simulink model "top_level_57_ALL_bergeron"  (R2025b)
settings: Solver=FixedStepDiscrete  StartTime=0.0  StopTime=50  FixedStep=Ts  RelTol=1e-3
undefined symbols (not defined in the file): DiscIntNeverNeededParam, droop, genTrip, idxGenTrip, idxSG_01, idxSMa, idxSMb, n_genP_pu, n_vRef_pu, noSG, noSM, Pref_lock, rateV, tagI, Ts, wref
libraries: simulink x4, ee_lib_for_power_systems x2, eeGeneralControl x1, eeSinusoidalMeasurementV2 x1
settings Model: SimulationMode=accelerator  Creator=gdudgeon  LastModifiedBy=gdudgeon
settings DataIOCC: SaveOutput=off  DSMLogging=off  InspectSignalLogs=on  SaveTime=off
settings ModelReferenceCC: UpdateModelReferenceTargets=AssumeUpToDate  ParallelModelReferenceMATLABWorkerInit=Copy Base Workspace

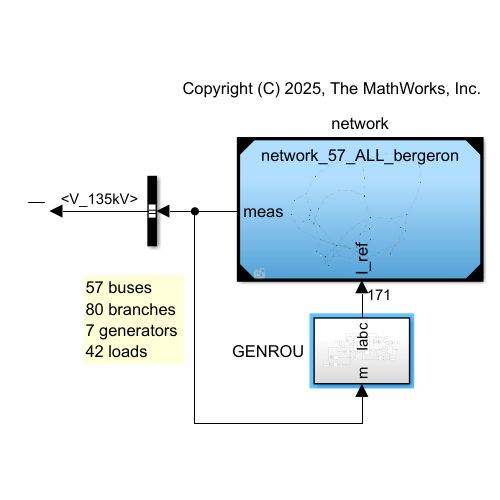
[thumbnail: Simulink's stored preview of the top-level diagram]
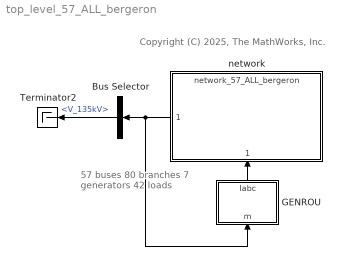
== system top_level_57_ALL_bergeron ==
  note: 57 buses
      | 80 branches
      | 7 generators
      | 42 loads
  note: Copyright (C) 2025, The MathWorks, Inc.
  Bus Selector : BusSelector  OutputSignals=V_135kV
  GENROU : Subsystem
  Terminator2 : Terminator
  network : ModelReference  ModelNameDialog=network_57_ALL_bergeron  ModelReferenceVersion=5.1
      settings: PortSchema="{\"entries\":[{\"content\":{\"sides\":[{\"content\":{\"connectorIds\":[\"Out1\"]},\"type\":\"ConnectorPlacement.EquallySpacedRectSide\",\"uuid\":\"a74df316-1767-4f8a-840d-17e03cd258f4\"},{\"content\":{\"side\":\"RIGHT\"},\"type\":\"ConnectorPlacement.EquallySpacedRectSide\",\"uuid\":\"1b3c021f-69ce-4b13-aefa-cee96e0614ce\"},{\"content\":{\"side\":\"TOP\"},\"type\":\"ConnectorPlacement.EquallySpacedRectSide\",\"uuid\":\"ae15f7f3-c1e2-4a2f-99df-e8d2d0ffd4ae\"},{\"content\":{\"connectorIds\":[\"In1\"],\"side\":\"BOTTOM\"},\"type\":\"ConnectorPlacement.EquallySpacedRectSide\",\"uuid\":\"649ce0cc-47ac-44c8-b67b-0ed46c10a575\"}]},\"type\":\"ConnectorPlacement.EquallySpacedConnector\",\"uuid\":\"f8de1fa7-a54d-42cb-bb68-f09d9f668e45\"}],\"packageUris\":[\"http://schema.mathworks.com/mf0/Connector/R2020b\"],\"version\":\"1.0\"}"
  wires:
  GENROU/1(Iabc) -> network/1
  network/1 -> Bus Selector/1, GENROU/1(m)
  Bus Selector/1 -> Terminator2/1  "<V_135kV>"

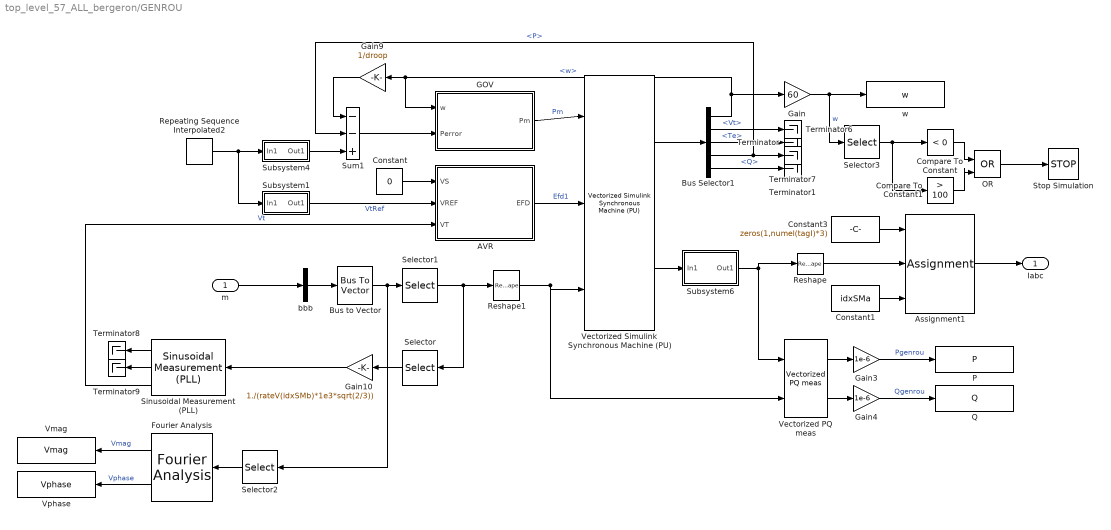
== system top_level_57_ALL_bergeron/GENROU ==
  m : Inport
  AVR : Subsystem  mask{K=500*ones(1,numel(idxSMb)), TE=0.05*ones(1,numel(idxSMb)), EMIN=0*ones(1,numel(idxSMb)), EMAX=4*ones(1,numel(idxSMb))}
      mask Display: disp('AVR')
  Assignment1 : Assignment  IndexOptions=Index vector (port)  Indices=1  OutputSizes=1
  Bus Selector1 : BusSelector  OutputSignals=w,Vt,Te,P,Q
  Bus to Vector : BusToVector
  Compare To Constant : simulink/Logic and Bit Operations/Compare To Constant  relop=<  const=0  OutDataTypeStr=boolean
  Compare To Constant1 : simulink/Logic and Bit Operations/Compare To Constant  relop=>  const=100  OutDataTypeStr=boolean
  Constant : Constant  Value=0  SampleTime=Ts
  Constant1 : Constant  Value=idxSMa  SampleTime=Ts
  Constant3 : Constant  Value=zeros(1,numel(tagI)*3)  SampleTime=Ts
  Fourier Analysis : eeGeneralControl/Fourier Analysis  f=freq  n=1  M0=1  Ph0=0  BufferSize=8192  Ts=Ts
      settings: LibrarySourceBlock=ee_sl_lib/General Control/Fourier Analysis
  GOV : Subsystem
      mask Display: disp('GOV')
  Gain : Gain  Gain=60
  Gain10 : Gain  Gain=1./(rateV(idxSMb)*1e3*sqrt(2/3))
  Gain3 : Gain  Gain=1e-6
  Gain4 : Gain  Gain=1e-6
  Gain9 : Gain  Gain=1/droop
  OR : Logic  Operator=OR  IconShape=distinctive  AllPortsSameDT=off  OutDataTypeStr=boolean
  P : ToWorkspace  VariableName=P  SaveFormat=Timeseries  SampleTime=Ts
  Q : ToWorkspace  VariableName=Q  SaveFormat=Timeseries  SampleTime=Ts
  Repeating Sequence Interpolated2 : simulink/Sources/Repeating Sequence Interpolated  OutValues=[0 0 1 1]  TimeValues=[0 0.2 1 110]  LookUpMeth=Interpolation-Use End Values  tsamp=Ts  OutMin=[]  OutMax=[]  OutDataTypeStr=double  OutputDataTypeScalingMode=double  OutDataType=fixdt(0,8)  OutScaling=2^-10
  Reshape : Reshape
  Reshape1 : Reshape  OutputDimensionality=Customize  OutputDimensions=[3,numel(idxSMb)]
  Selector : Selector  InputPortWidth=numel(idxSMb)*3  IndexOptions=Index vector (dialog)  Indices=1:3:numel(idxSMb)*3  OutputSizes=1
  Selector1 : Selector  InputPortWidth=numel(tagI)*3  IndexOptions=Index vector (dialog)  Indices=idxSMa  OutputSizes=1
  Selector2 : Selector  InputPortWidth=57*3  IndexOptions=Index vector (dialog)  Indices=1:3:(57*3)  OutputSizes=1
  Selector3 : Selector  InputPortWidth=noSM  IndexOptions=Index vector (dialog)  Indices=1  OutputSizes=1
  Sinusoidal Measurement (PLL) : eeSinusoidalMeasurementV2/Sinusoidal Measurement (PLL)  Ki_PD=1000  Kp_LF=400  Ki_LF=20000  F0=60  Theta0=0  Mag0=0  Ts=Ts
      settings: LibrarySourceBlock=|
      | ee_sl_lib/Measurements/Sinusoidal Measurement
      | (PLL)
  Stop Simulation : Stop
  Subsystem1 : Subsystem
  Subsystem4 : Subsystem
  Subsystem6 : Subsystem  mask{tn=idxGenTrip}
      mask prompts: tn "Generator index"
      mask Display: disp('TRIP')
  Sum1 : Sum  Inputs=--+
  Terminator{,1,6..9} (6 alike) : Terminator
  Vectorized PQ meas : ee_lib_for_power_systems/Sense and Measure/Vectorized PQ meas  SystemSampleTime=-1  VariantActivationTime=update diagram  EmptyChoice=off  PassThrough=off  PassThroughVariantControl=(default)  EmptyChoiceVariantControl=(default)  AllowFlexibleInterface=on  Latency=0  AutoFrameSizeCalculation=off
      settings: LibrarySourceBlock=|
      | sps_lib/Sensors and Measurements/Power
      | (3ph, Instantaneous)
  Vectorized Simulink Synchronous Machine (PU) : ee_lib_for_power_systems/Electromechanical Machines/Vectorized Simulink Synchronous Machine (PU)  Pnom=nomP_SM  Vnom=rateV(idxSMb)*1e3  fnom=60*ones(1,noSM)  NPP=4*ones(1,noSM)  Ra=0.05*ones(1,noSM)  Xl=0.1*ones(1,noSM)  Xd=1.5*ones(1,noSM)  Xq=1.4*ones(1,noSM)  Xdp=0.4*ones(1,noSM)  Xqp=0.5*ones(1,noSM)  Xdpp=0.25*ones(1,noSM)  Xqpp=0.25*ones(1,noSM)  Tdop=5*ones(1,noSM)  Tqop=1.5*ones(1,noSM)  Tdopp=0.6*ones(1,noSM)  Tqopp=0.06*ones(1,noSM)  H=4*ones(1,noSM)  D=zeros(1,noSM)  SatX=SatX  xVec=xVec  no_gens=noSM
      settings: SourceProductName=Support Library for Power Systems
  Vmag : ToWorkspace  VariableName=Vmag  SaveFormat=Timeseries  SampleTime=Ts
  Vphase : ToWorkspace  VariableName=Vphase  SaveFormat=Timeseries  SampleTime=Ts
  bbb : BusSelector  OutputSignals=V_135kV  OutputAsBus=on
  w : ToWorkspace  VariableName=w  SaveFormat=Timeseries  SampleTime=Ts
  Iabc : Outport
  wires:
  Gain3/1 -> P/1  "Pgenrou"
  Vectorized PQ meas/1 -> Gain3/1
  Vectorized PQ meas/2 -> Gain4/1
  Gain4/1 -> Q/1  "Qgenrou"
  Bus Selector1/3 -> Terminator/1  "<Te>"
  Vectorized Simulink Synchronous Machine (PU)/1 -> Bus Selector1/1
  Reshape1/1 -> Vectorized Simulink Synchronous Machine (PU)/3, Vectorized PQ meas/2
  Vectorized Simulink Synchronous Machine (PU)/2 -> Subsystem6/1(In1)
  Constant3/1 -> Assignment1/1
  Constant1/1 -> Assignment1/3
  Assignment1/1 -> Iabc/1
  Repeating Sequence Interpolated2/1 -> Subsystem1/1(In1), Subsystem4/1(In1)
  Reshape/1 -> Assignment1/2
  Subsystem6/1(Out1) -> Vectorized PQ meas/1, Reshape/1
  Bus Selector1/5 -> Terminator1/1  "<Q>"
  Bus Selector1/2 -> Terminator6/1  "<Vt>"
  Bus Selector1/1 -> Gain/1, GOV/1(w), Gain9/1  "<w>"
  Bus Selector1/4 -> Sum1/2, Terminator7/1  "<P>"
  Sum1/1 -> GOV/2(Perror)
  Selector/1 -> Gain10/1
  Sinusoidal Measurement (PLL)/3 -> AVR/3(VT)  "Vt"
  Gain10/1 -> Sinusoidal Measurement (PLL)/1
  Sinusoidal Measurement (PLL)/1 -> Terminator8/1
  Sinusoidal Measurement (PLL)/2 -> Terminator9/1
  Gain9/1 -> Sum1/1
  Subsystem1/1(Out1) -> AVR/2(VREF)  "VtRef"
  Subsystem4/1(Out1) -> Sum1/3
  Gain/1 -> Selector3/1, w/1  "w"
  Constant/1 -> AVR/1(VS)
  m/1 -> bbb/1
  bbb/1 -> Bus to Vector/1
  Selector1/1 -> Selector/1, Reshape1/1
  GOV/1(Pm) -> Vectorized Simulink Synchronous Machine (PU)/1  "Pm"
  AVR/1(EFD) -> Vectorized Simulink Synchronous Machine (PU)/2  "Efd1"
  Fourier Analysis/1 -> Vmag/1  "Vmag"
  Fourier Analysis/2 -> Vphase/1  "Vphase"
  Selector2/1 -> Fourier Analysis/1
  Bus to Vector/1 -> Selector2/1, Selector1/1
  Selector3/1 -> Compare To Constant1/1, Compare To Constant/1
  Compare To Constant/1 -> OR/1
  Compare To Constant1/1 -> OR/2
  OR/1 -> Stop Simulation/1

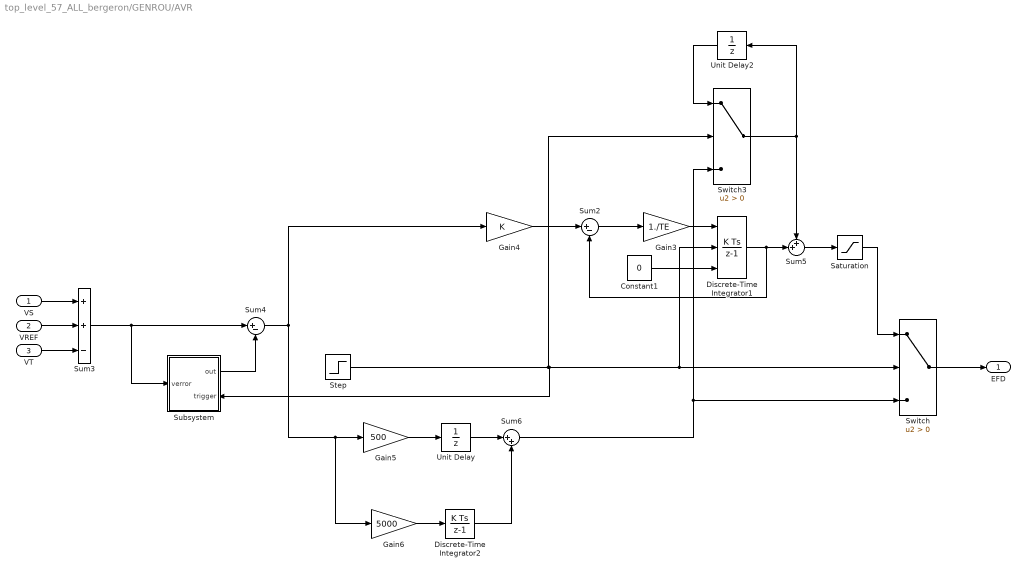
== system top_level_57_ALL_bergeron/GENROU/AVR ==
  VS : Inport
  VREF : Inport  Port=2
  VT : Inport  Port=3
  Constant1 : Constant  Value=0  SampleTime=Ts
  Discrete-Time Integrator1 : DiscreteIntegrator  ExternalReset=rising  InitialConditionSource=external  SampleTime=Ts  UpperSaturationLimit=EMAX  LowerSaturationLimit=EMIN  ICPrevOutput=DiscIntNeverNeededParam  ICPrevScaledInput=DiscIntNeverNeededParam
  Discrete-Time Integrator2 : DiscreteIntegrator  SampleTime=-1  ICPrevOutput=DiscIntNeverNeededParam  ICPrevScaledInput=DiscIntNeverNeededParam
  Gain3 : Gain  Gain=1./TE
  Gain4 : Gain  Gain=K
  Gain5 : Gain  Gain=500
  Gain6 : Gain  Gain=5000
  Saturation : Saturate  UpperLimit=EMAX  LowerLimit=EMIN
  Step : Step  Time=Pref_lock  SampleTime=Ts
  Subsystem : Subsystem
      settings: PortSchema="{\"entries\":[{\"content\":{\"sides\":[{\"content\":{\"connectorIds\":[\"In1\"]},\"type\":\"ConnectorPlacement.EquallySpacedRectSide\",\"uuid\":\"fcea7782-709e-438a-a641-262ec3f31354\"},{\"content\":{\"connectorIds\":[\"Out1\",\"In2\"],\"side\":\"RIGHT\"},\"type\":\"ConnectorPlacement.EquallySpacedRectSide\",\"uuid\":\"9571ea79-f1f3-4aec-b926-22759d29ebce\"},{\"content\":{\"side\":\"TOP\"},\"type\":\"ConnectorPlacement.EquallySpacedRectSide\",\"uuid\":\"bf0a6030-28c1-4408-9c1d-af564ece2abc\"}]},\"type\":\"ConnectorPlacement.EquallySpacedConnector\",\"uuid\":\"5fd903bf-193d-421d-8000-bea997fdfc71\"}],\"packageUris\":[\"http://schema.mathworks.com/mf0/Connector/R2020b\"],\"version\":\"1.0\"}"
  Sum2 : Sum  Inputs=|+-
  Sum3 : Sum  Inputs=++-
  Sum4 : Sum  Inputs=|+-
  Sum5 : Sum  Inputs=++|
  Sum6 : Sum  Inputs=|++
  Switch : Switch  Criteria=u2 > Threshold  SaturateOnIntegerOverflow=off  InputSameDT=off
  Switch3 : Switch  Criteria=u2 > Threshold  SaturateOnIntegerOverflow=off  InputSameDT=off
  Unit Delay : UnitDelay  SampleTime=Ts  HasFrameUpgradeWarning=on
  Unit Delay2 : UnitDelay  SampleTime=Ts  HasFrameUpgradeWarning=on
  EFD : Outport
  wires:
  VS/1 -> Sum3/1
  VREF/1 -> Sum3/2
  VT/1 -> Sum3/3
  Gain4/1 -> Sum2/1
  Sum2/1 -> Gain3/1
  Gain3/1 -> Discrete-Time Integrator1/1
  Switch/1 -> EFD/1
  Sum6/1 -> Switch3/3, Switch/3
  Step/1 -> Discrete-Time Integrator1/2, Switch/2, Subsystem/2(trigger), Switch3/2
  Discrete-Time Integrator1/1 -> Sum2/2, Sum5/2
  Sum5/1 -> Saturation/1
  Switch3/1 -> Unit Delay2/1, Sum5/1
  Unit Delay2/1 -> Switch3/1
  Constant1/1 -> Discrete-Time Integrator1/3
  Gain5/1 -> Unit Delay/1
  Saturation/1 -> Switch/1
  Gain6/1 -> Discrete-Time Integrator2/1
  Discrete-Time Integrator2/1 -> Sum6/2
  Sum4/1 -> Gain4/1, Gain5/1, Gain6/1
  Unit Delay/1 -> Sum6/1
  Subsystem/1(out) -> Sum4/2
  Sum3/1 -> Subsystem/1(verror), Sum4/1

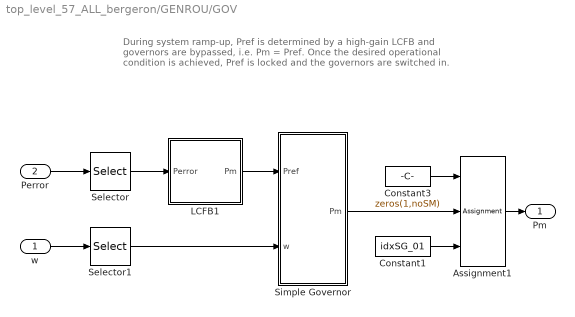
== system top_level_57_ALL_bergeron/GENROU/GOV ==
  note: During system ramp-up, Pref is determined by a high-gain LCFB and governors are bypassed, i.e. Pm = Pref.
      |
      | Once the desired operational condition is achieved, Pref is locked and the governors are switched in.
  w : Inport
  Perror : Inport  Port=2
  Assignment1 : Assignment  IndexOptions=Index vector (port)  Indices=1  OutputSizes=1
  Constant1 : Constant  Value=idxSG_01  SampleTime=Ts
  Constant3 : Constant  Value=zeros(1,noSM)  SampleTime=Ts
  LCFB1 : Subsystem
  Selector : Selector  InputPortWidth=noSM  IndexOptions=Index vector (dialog)  Indices=idxSG_01  OutputSizes=1
  Selector1 : Selector  InputPortWidth=noSM  IndexOptions=Index vector (dialog)  Indices=idxSG_01  OutputSizes=1
  Simple Governor : Subsystem  mask{R=0.2*ones(1,noSG), T1=3*ones(1,noSG), P_MAX=2*ones(1,noSG), P_MIN=0*ones(1,noSG)}
  Pm : Outport
  wires:
  LCFB1/1(Pm) -> Simple Governor/1(Pref)
  Perror/1 -> Selector/1
  w/1 -> Selector1/1
  Simple Governor/1(Pm) -> Assignment1/2
  Constant3/1 -> Assignment1/1
  Constant1/1 -> Assignment1/3
  Assignment1/1 -> Pm/1
  Selector/1 -> LCFB1/1(Perror)
  Selector1/1 -> Simple Governor/2(w)

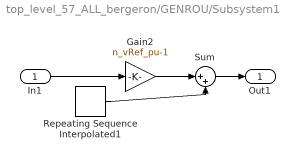
== system top_level_57_ALL_bergeron/GENROU/Subsystem1 ==
  In1 : Inport
  Gain2 : Gain  Gain=n_vRef_pu-1
  Repeating Sequence Interpolated1 : simulink/Sources/Repeating Sequence Interpolated  OutValues=[0 0 1 1]*1  TimeValues=[0 0.05 0.1 110]  LookUpMeth=Interpolation-Use End Values  tsamp=Ts  OutMin=[]  OutMax=[]  OutDataTypeStr=double  OutputDataTypeScalingMode=double  OutDataType=fixdt(0,8)  OutScaling=2^-10
  Sum : Sum  Inputs=|++
  Out1 : Outport
  wires:
  Gain2/1 -> Sum/1
  Repeating Sequence Interpolated1/1 -> Sum/2
  Sum/1 -> Out1/1
  In1/1 -> Gain2/1

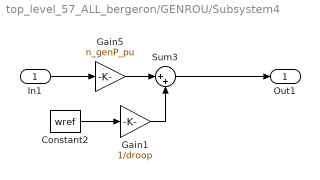
== system top_level_57_ALL_bergeron/GENROU/Subsystem4 ==
  In1 : Inport
  Constant2 : Constant  Value=wref  VectorParams1D=off  SampleTime=Ts
  Gain1 : Gain  Gain=1/droop
  Gain5 : Gain  Gain=n_genP_pu
  Sum3 : Sum  Inputs=|++
  Out1 : Outport
  wires:
  Sum3/1 -> Out1/1
  Gain1/1 -> Sum3/2
  Gain5/1 -> Sum3/1
  In1/1 -> Gain5/1
  Constant2/1 -> Gain1/1

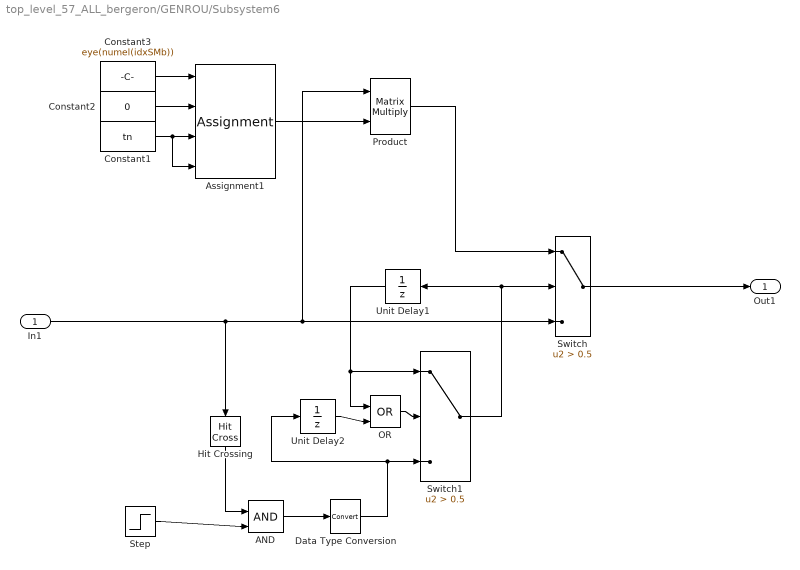
== system top_level_57_ALL_bergeron/GENROU/Subsystem6 ==
  In1 : Inport
  AND : Logic  IconShape=distinctive  AllPortsSameDT=off  OutDataTypeStr=boolean
  Assignment1 : Assignment  NumberOfDimensions=2  IndexOptions=Index vector (port),Index vector (port)  Indices=1,1  OutputSizes=1,1
  Constant1 : Constant  Value=tn  SampleTime=Ts
  Constant2 : Constant  Value=0  SampleTime=Ts
  Constant3 : Constant  Value=eye(numel(idxSMb))  VectorParams1D=off  SampleTime=Ts
  Data Type Conversion : DataTypeConversion  SaturateOnIntegerOverflow=off  RndMeth=Floor
  Hit Crossing : HitCross
  OR : Logic  Operator=OR  IconShape=distinctive  AllPortsSameDT=off  OutDataTypeStr=boolean
  Product : Product  Multiplication=Matrix(*)
  Step : Step  Time=genTrip  SampleTime=Ts
  Switch : Switch  Criteria=u2 > Threshold  Threshold=0.5  SaturateOnIntegerOverflow=off  InputSameDT=off
  Switch1 : Switch  Criteria=u2 > Threshold  Threshold=0.5  SaturateOnIntegerOverflow=off  InputSameDT=off
  Unit Delay1 : UnitDelay  SampleTime=-1  HasFrameUpgradeWarning=on
  Unit Delay2 : UnitDelay  SampleTime=-1  HasFrameUpgradeWarning=on
  Out1 : Outport
  wires:
  Step/1 -> AND/2
  Switch1/1 -> Unit Delay1/1, Switch/2
  Data Type Conversion/1 -> Unit Delay2/1, Switch1/3
  Unit Delay1/1 -> OR/1, Switch1/1
  OR/1 -> Switch1/2
  Product/1 -> Switch/1
  Hit Crossing/1 -> AND/1
  Switch/1 -> Out1/1
  AND/1 -> Data Type Conversion/1
  Unit Delay2/1 -> OR/2
  In1/1 -> Hit Crossing/1, Product/1, Switch/3
  Constant1/1 -> Assignment1/4, Assignment1/3
  Constant3/1 -> Assignment1/1
  Constant2/1 -> Assignment1/2
  Assignment1/1 -> Product/2

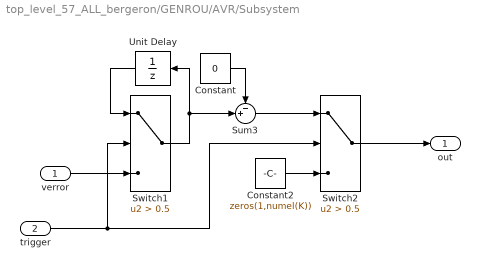
== system top_level_57_ALL_bergeron/GENROU/AVR/Subsystem ==
  verror : Inport
  trigger : Inport  Port=2
  Constant : Constant  Value=0  SampleTime=Ts
  Constant2 : Constant  Value=zeros(1,numel(K))  SampleTime=Ts
  Sum3 : Sum  Inputs=-+|
  Switch1 : Switch  Criteria=u2 > Threshold  Threshold=0.5  SaturateOnIntegerOverflow=off  InputSameDT=off
  Switch2 : Switch  Criteria=u2 > Threshold  Threshold=0.5  SaturateOnIntegerOverflow=off  InputSameDT=off
  Unit Delay : UnitDelay  SampleTime=Ts  HasFrameUpgradeWarning=on
  out : Outport
  wires:
  verror/1 -> Switch1/3
  Switch1/1 -> Sum3/2, Unit Delay/1
  Constant2/1 -> Switch2/3
  trigger/1 -> Switch2/2, Switch1/2
  Unit Delay/1 -> Switch1/1
  Sum3/1 -> Switch2/1
  Switch2/1 -> out/1
  Constant/1 -> Sum3/1

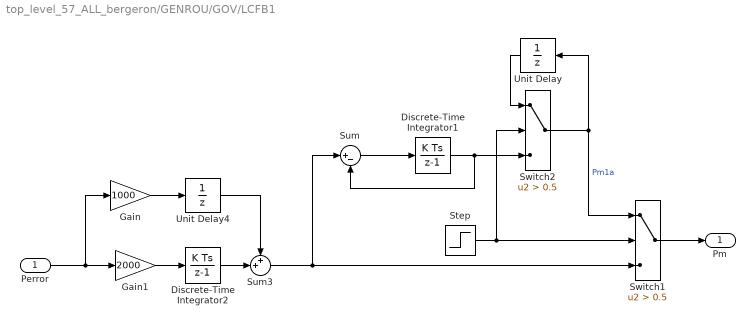
== system top_level_57_ALL_bergeron/GENROU/GOV/LCFB1 ==
  Perror : Inport
  Discrete-Time Integrator1 : DiscreteIntegrator  gainval=10  SampleTime=Ts  LowerSaturationLimit=0  ICPrevOutput=DiscIntNeverNeededParam  ICPrevScaledInput=DiscIntNeverNeededParam
  Discrete-Time Integrator2 : DiscreteIntegrator  gainval=1  SampleTime=Ts  LimitOutput=on  LowerSaturationLimit=0  ICPrevOutput=DiscIntNeverNeededParam  ICPrevScaledInput=DiscIntNeverNeededParam
  Gain : Gain  Gain=1000
  Gain1 : Gain  Gain=2000
  Step : Step  Time=Pref_lock  SampleTime=Ts
  Sum : Sum  Inputs=|+-
  Sum3 : Sum  Inputs=++|
  Switch1 : Switch  Criteria=u2 > Threshold  Threshold=0.5  SaturateOnIntegerOverflow=off  InputSameDT=off
  Switch2 : Switch  Criteria=u2 > Threshold  Threshold=0.5  SaturateOnIntegerOverflow=off  InputSameDT=off
  Unit Delay : UnitDelay  SampleTime=Ts  HasFrameUpgradeWarning=on
  Unit Delay4 : UnitDelay  SampleTime=Ts  HasFrameUpgradeWarning=on
  Pm : Outport
  wires:
  Perror/1 -> Gain/1, Gain1/1
  Unit Delay4/1 -> Sum3/1
  Discrete-Time Integrator2/1 -> Sum3/2
  Switch1/1 -> Pm/1
  Step/1 -> Switch2/2, Switch1/2
  Gain/1 -> Unit Delay4/1
  Gain1/1 -> Discrete-Time Integrator2/1
  Discrete-Time Integrator1/1 -> Switch2/3, Sum/2
  Sum/1 -> Discrete-Time Integrator1/1
  Sum3/1 -> Switch1/3, Sum/1
  Switch2/1 -> Switch1/1, Unit Delay/1  "Pm1a"
  Unit Delay/1 -> Switch2/1

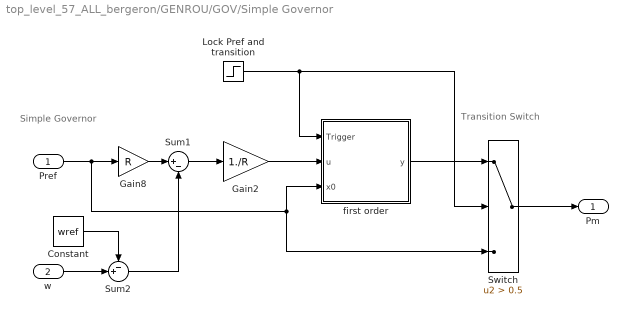
== system top_level_57_ALL_bergeron/GENROU/GOV/Simple Governor ==
  note: Transition Switch
  note: Simple Governor
  Pref : Inport
  w : Inport  Port=2
  Constant : Constant  Value=wref  SampleTime=Ts
  Gain2 : Gain  Gain=1./R
  Gain8 : Gain  Gain=R
  Lock Pref and transition : Step  Time=Pref_lock  SampleTime=Ts
  Sum1 : Sum  Inputs=|+-
  Sum2 : Sum  Inputs=-+|
  Switch : Switch  Criteria=u2 > Threshold  Threshold=0.5  SaturateOnIntegerOverflow=off  InputSameDT=off
  first order : Subsystem
      mask Display: fprintf('1\n------------\n1 + T1s');
  Pm : Outport
  wires:
  Sum1/1 -> Gain2/1
  Pref/1 -> Switch/3, first order/3(x0), Gain8/1
  Switch/1 -> Pm/1
  Lock Pref and transition/1 -> first order/1(Trigger), Switch/2
  first order/1(y) -> Switch/1
  Constant/1 -> Sum2/1
  Sum2/1 -> Sum1/2
  Gain8/1 -> Sum1/1
  Gain2/1 -> first order/2(u)
  w/1 -> Sum2/2

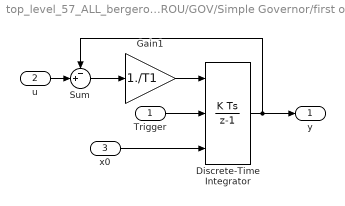
== system top_level_57_ALL_bergeron/GENROU/GOV/Simple Governor/first order ==
  Trigger : Inport
  u : Inport  Port=2
  x0 : Inport  Port=3
  Discrete-Time Integrator : DiscreteIntegrator  ExternalReset=rising  InitialConditionSource=external  SampleTime=Ts  LimitOutput=on  UpperSaturationLimit=P_MAX  LowerSaturationLimit=P_MIN  ICPrevOutput=DiscIntNeverNeededParam  ICPrevScaledInput=DiscIntNeverNeededParam
  Gain1 : Gain  Gain=1./T1
  Sum : Sum  Inputs=-+|
  y : Outport
  wires:
  Trigger/1 -> Discrete-Time Integrator/2
  u/1 -> Sum/2
  Sum/1 -> Gain1/1
  x0/1 -> Discrete-Time Integrator/3
  Discrete-Time Integrator/1 -> y/1, Sum/1
  Gain1/1 -> Discrete-Time Integrator/1
